simulink model "eval_pf"  (R2026a)
settings: Solver=FixedStepAuto  StopTime=1000
undefined symbols (not defined in the file): pf_param, plant_param, r_param
libraries: lib_sensors x3, lib_plant x1
settings Model: Creator=alessandro-nardin  LastModifiedBy=fiore
settings RTWCC: Toolchain=Microsoft Visual C++ 2022 v17.0 | nmake (64-bit Windows)

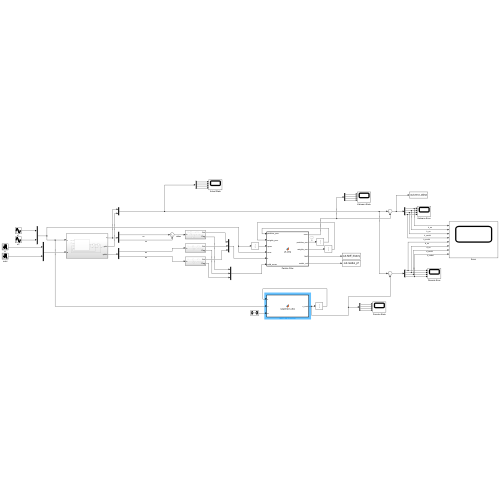
[thumbnail: Simulink's stored preview of the top-level diagram]
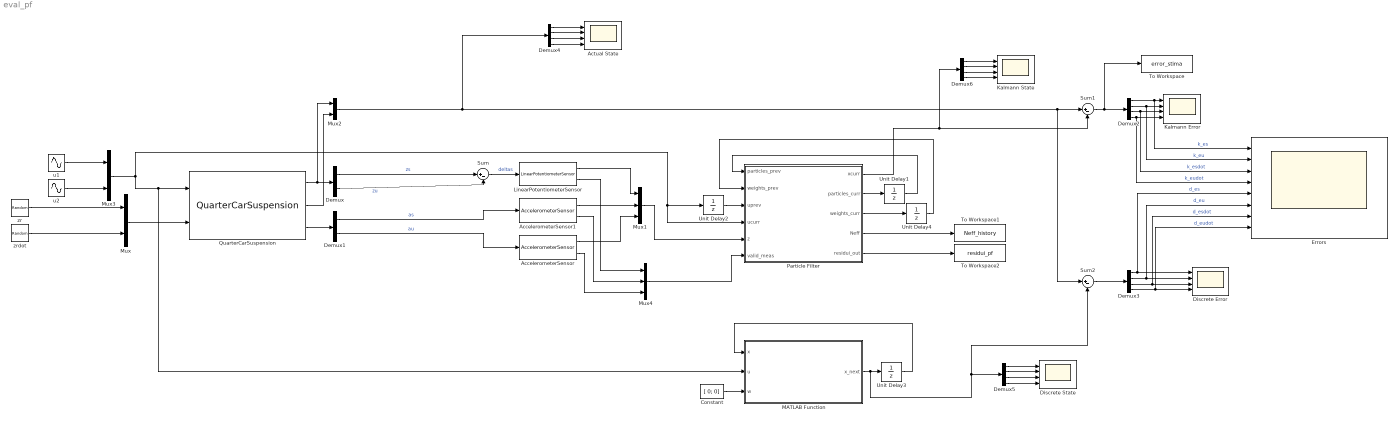
== system eval_pf ==
  AccelerometerSensor : lib_sensors/AccelerometerSensor  SystemSampleTime=-1  VariantActivationTime=update diagram  EmptyChoice=off  PassThrough=off  PassThroughVariantControl=(default)  EmptyChoiceVariantControl=(default)  AllowFlexibleInterface=on  Latency=0  AutoFrameSizeCalculation=off
  AccelerometerSensor1 : lib_sensors/AccelerometerSensor  SystemSampleTime=-1  VariantActivationTime=update diagram  EmptyChoice=off  PassThrough=off  PassThroughVariantControl=(default)  EmptyChoiceVariantControl=(default)  AllowFlexibleInterface=on  Latency=0  AutoFrameSizeCalculation=off
  Actual State : Scope  NumInputPorts=4
      settings: ActiveDisplayYMinimum=-13.406936930450598  ActiveDisplayYMaximum=16.431517639223237  DataLoggingVariableName=ScopeData2
  Constant : Constant  Value=[ 0; 0]
  Demux : Demux  Outputs=2
  Demux1 : Demux  Outputs=2
  Demux{2..6} (5 alike) : Demux
  Discrete Error : Scope  NumInputPorts=4
      settings: ActiveDisplayYMinimum=-0.13461336894615539  ActiveDisplayYMaximum=0.12972172873522425
  Discrete State : Scope  NumInputPorts=4
      settings: ActiveDisplayYMinimum=-16.662431963356159  ActiveDisplayYMaximum=16.863664846001409  DataLoggingVariableName=ScopeData3
  Errors : Scope  NumInputPorts=8
      settings: ActiveDisplayYMinimum=-0.10887280087153245  ActiveDisplayYMaximum=0.11805338023274278  DataLoggingVariableName=ScopeData5
  Kalmann Error : Scope  NumInputPorts=4
      settings: ActiveDisplayYMinimum=-2.0556820969120144  ActiveDisplayYMaximum=2.2410085599470091
  Kalmann State : Scope  NumInputPorts=4
      settings: ActiveDisplayYMinimum=-12.347879763067127  ActiveDisplayYMaximum=15.301795380492928  DataLoggingVariableName=ScopeData4
  LinearPotentiometerSensor : lib_sensors/LinearPotentiometerSensor  SystemSampleTime=-1  VariantActivationTime=update diagram  EmptyChoice=off  PassThrough=off  PassThroughVariantControl=(default)  EmptyChoiceVariantControl=(default)  AllowFlexibleInterface=on  Latency=0  AutoFrameSizeCalculation=off
  MATLAB Function : MATLAB Function  TreatAsAtomicUnit=on
  Mux : Mux  Inputs=2
  Mux1 : Mux  Inputs=3
  Mux2 : Mux  Inputs=2
  Mux3 : Mux  Inputs=2
  Mux4 : Mux  Inputs=3
  Particle Filter : MATLAB Function  TreatAsAtomicUnit=on
  QuarterCarSuspension : lib_plant/QuarterCarSuspension  SystemSampleTime=-1  VariantActivationTime=update diagram  EmptyChoice=off  PassThrough=off  PassThroughVariantControl=(default)  EmptyChoiceVariantControl=(default)  AllowFlexibleInterface=on  Latency=0  AutoFrameSizeCalculation=off
      settings: SourceProductName=Lib Plant
  Sum : Sum  Inputs=|+-
  Sum1 : Sum  Inputs=|+-
  Sum2 : Sum  Inputs=|+-
  To Workspace : ToWorkspace  VariableName=error_stima  SaveFormat=Timeseries  SampleTime=-1
  To Workspace1 : ToWorkspace  VariableName=Neff_history  SaveFormat=Timeseries  SampleTime=-1
  To Workspace2 : ToWorkspace  VariableName=residui_pf  SaveFormat=Timeseries  SampleTime=-1
  Unit Delay1 : UnitDelay  InitialCondition=pf_param.particles_init  SampleTime=pf_param.sample_t
  Unit Delay2 : UnitDelay  InitialCondition=[ 0; 0]  SampleTime=pf_param.sample_t
  Unit Delay3 : UnitDelay  InitialCondition=pf_param.x_init  SampleTime=-1
  Unit Delay4 : UnitDelay  InitialCondition=pf_param.weights_init  SampleTime=pf_param.sample_t
  u1 : Sin  Amplitude=943  Frequency=0.5  Phase=0.2  SampleTime=0
  u2 : Sin  Amplitude=2000  Phase=1  SampleTime=0
  zr : RandomNumber  Variance=r_param.rz_var  Seed=3245  SampleTime=0
  zrdot : RandomNumber  Variance=r_param.rzdot_var  Seed=213  SampleTime=0
  wires:
  QuarterCarSuspension/1 -> Demux/1, Mux2/1
  Demux/1 -> Sum/1  "zs"
  Demux/2 -> Sum/2  "zu"
  Sum/1 -> LinearPotentiometerSensor/1  "deltas"
  Demux1/2 -> AccelerometerSensor/1  "au"
  QuarterCarSuspension/3 -> Demux1/1
  Demux1/1 -> AccelerometerSensor1/1  "as"
  Mux/1 -> QuarterCarSuspension/2
  Particle Filter/2(particles_curr) -> Unit Delay1/1
  Unit Delay1/1 -> Particle Filter/1(particles_prev)
  Mux3/1 -> QuarterCarSuspension/1, MATLAB Function/2(u), Particle Filter/4(ucurr), Unit Delay2/1
  Unit Delay2/1 -> Particle Filter/3(uprev)
  AccelerometerSensor1/1 -> Mux1/2
  Mux1/1 -> Particle Filter/5(z)
  zr/1 -> Mux/1
  zrdot/1 -> Mux/2
  u1/1 -> Mux3/1
  u2/1 -> Mux3/2
  Unit Delay3/1 -> MATLAB Function/1(x)
  Constant/1 -> MATLAB Function/3(w)
  QuarterCarSuspension/2 -> Mux2/2
  Sum1/1 -> To Workspace/1, Demux2/1
  Demux2/1 -> Errors/1, Kalmann Error/1  "k_es"
  Demux2/2 -> Errors/2, Kalmann Error/2  "k_eu"
  Demux2/3 -> Errors/3, Kalmann Error/3  "k_esdot"
  Demux2/4 -> Errors/4, Kalmann Error/4  "k_eudot"
  Sum2/1 -> Demux3/1
  Demux3/4 -> Errors/8, Discrete Error/4  "d_eudot"
  Demux3/2 -> Errors/6, Discrete Error/2  "d_eu"
  Demux3/1 -> Errors/5, Discrete Error/1  "d_es"
  Demux3/3 -> Errors/7, Discrete Error/3  "d_esdot"
  Demux4/4 -> Actual State/4
  Mux2/1 -> Demux4/1, Sum2/1, Sum1/1
  Demux4/2 -> Actual State/2
  Demux4/3 -> Actual State/3
  Demux4/1 -> Actual State/1
  Demux5/4 -> Discrete State/4
  MATLAB Function/1(x_next) -> Sum2/2, Demux5/1, Unit Delay3/1
  Demux5/2 -> Discrete State/2
  Demux5/3 -> Discrete State/3
  Demux5/1 -> Discrete State/1
  Demux6/4 -> Kalmann State/4
  Particle Filter/1(xcurr) -> Sum1/2, Demux6/1
  Demux6/2 -> Kalmann State/2
  Demux6/3 -> Kalmann State/3
  Demux6/1 -> Kalmann State/1
  AccelerometerSensor/1 -> Mux1/3
  Mux4/1 -> Particle Filter/6(valid_meas)
  LinearPotentiometerSensor/2 -> Mux4/1
  AccelerometerSensor1/2 -> Mux4/2
  AccelerometerSensor/2 -> Mux4/3
  LinearPotentiometerSensor/1 -> Mux1/1
  Particle Filter/3(weights_curr) -> Unit Delay4/1
  Unit Delay4/1 -> Particle Filter/2(weights_prev)
  Particle Filter/4(Neff) -> To Workspace1/1
  Particle Filter/5(residui_out) -> To Workspace2/1

== matlab function eval_pf/MATLAB Function ==
  settings: updateMethod=DISCRETE  sampleTime=pf_param.sample_t
  data: x input; u input; x_next output size=[ 4 1 ]; w input; plant_param parameter; pf_param parameter
function x_next = suspension_dics( x, u, w, plant_param, pf_param)
x_next = suspension_f_dics_euler( x, u, w, plant_param, pf_param.sample_t);

== matlab function eval_pf/Particle Filter ==
  settings: updateMethod=DISCRETE  sampleTime=pf_param.sample_t
  data: particles_prev input; weights_prev input; uprev input; ucurr input; z input; plant_param parameter; pf_param parameter; xcurr output; particles_curr output; weights_curr output; valid_meas input; Neff output; residui_out output
function [xcurr, particles_curr, weights_curr, Neff, residui_out] = pf_step(particles_prev, weights_prev, uprev, ucurr, z, plant_param, pf_param, valid_meas)    % Simulink prenderà plant_param e pf_param direttamente dal workspace
    [xcurr, particles_curr, weights_curr, Neff, residui_out] = pf_step(particles_prev, weights_prev, uprev, ucurr, z, plant_param, pf_param, valid_meas);
end
